simulink model "usmc2"  (R2020b)
settings: Solver=VariableStepAuto  StartTime=0.0  StopTime=10  RelTol=1e-3
settings Model: Creator=Lenovo  LastModifiedBy=Lenovo

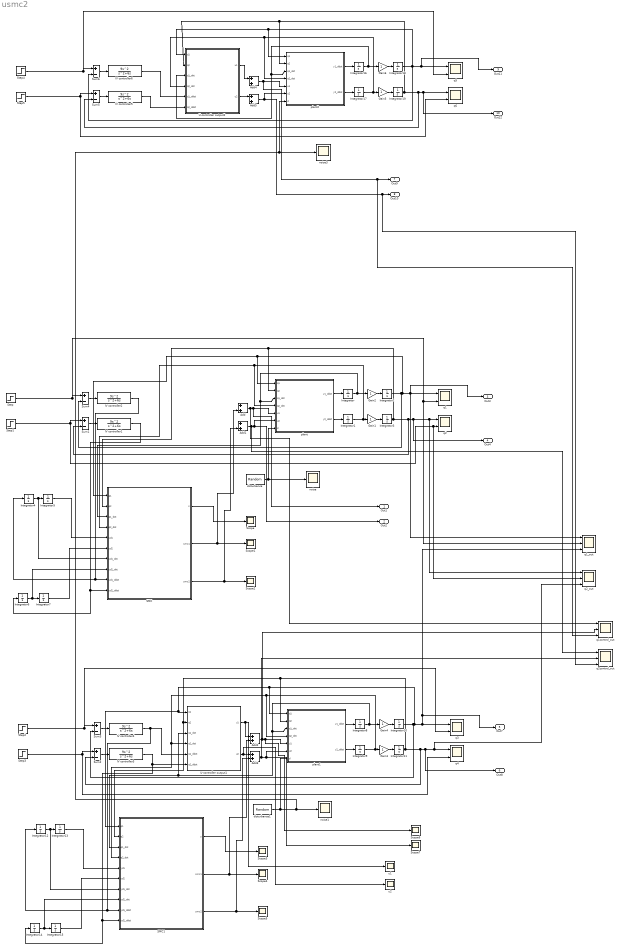
== system usmc2 ==
  Add{,1..5} (6 alike) : Sum
  Gain{1..6} (6 alike) : Gain
  IV controller{1..6} (6 alike) : TransferFcn  Numerator=[9 0 0]  Denominator=[1 6 0]
  Integrator{,1..19} (20 alike) : Integrator
  SMC : MATLAB Function  TreatAsAtomicUnit=on
  SMC1 : MATLAB Function  TreatAsAtomicUnit=on
  Scope{,1..7} (8 alike) : Scope
  Step : Step  After=3  SampleTime=0.001
  Step1 : Step  After=2  SampleTime=0.001
  Step2 : Step  After=3  SampleTime=0.001
  Step3 : Step  After=2  SampleTime=0.001
  Step4 : Step  After=3  SampleTime=0.001
  Step5 : Step  After=2  SampleTime=0.001
  Sum{1..6} (6 alike) : Sum  Inputs=|+-
  U-controller output1 : MATLAB Function  TreatAsAtomicUnit=on
  U-controller output2 : MATLAB Function  TreatAsAtomicUnit=on
  disturbance : UniformRandomNumber  Minimum=-10  Maximum=10  SampleTime=0.01
  disturbance1 : UniformRandomNumber  Minimum=-10  Maximum=10  SampleTime=0.01
  noise : Scope
  noise1 : Scope
  noise3 : Scope
  plant : MATLAB Function  TreatAsAtomicUnit=on
  plant1 : MATLAB Function  TreatAsAtomicUnit=on
  plant2 : MATLAB Function  TreatAsAtomicUnit=on
  q{1..6} (6 alike) : Scope  NumInputPorts=2
  q1_out : Scope  NumInputPorts=3
  q1control_out : Scope  NumInputPorts=3
  q2_out : Scope  NumInputPorts=3
  q2control_out : Scope  NumInputPorts=3
  u1 : Scope
  u2 : Scope
  Out1 : Outport  VectorParamsAs1DForOutWhenUnconnected=off
  Out2 : Outport  Port=2  VectorParamsAs1DForOutWhenUnconnected=off
  Out3 : Outport  Port=3  VectorParamsAs1DForOutWhenUnconnected=off
  Out4 : Outport  Port=4  VectorParamsAs1DForOutWhenUnconnected=off
  Out7 : Outport  Port=5  VectorParamsAs1DForOutWhenUnconnected=off
  Out8 : Outport  Port=6  VectorParamsAs1DForOutWhenUnconnected=off
  Out9 : Outport  Port=7  VectorParamsAs1DForOutWhenUnconnected=off
  Out10 : Outport  Port=8  VectorParamsAs1DForOutWhenUnconnected=off
  Out11 : Outport  Port=9  VectorParamsAs1DForOutWhenUnconnected=off
  Out12 : Outport  Port=10  VectorParamsAs1DForOutWhenUnconnected=off
  wires:
  Add5/1 -> q2control_out/3, Out10/1, plant2/6(u2)
  Integrator8/1 -> Gain4/1, SMC1/3(q1_dot), U-controller output1/3(q1_dot), plant1/3(q1_dot)
  Integrator16/1 -> Gain6/1, U-controller output2/3(q1_dot), plant2/3(q1_dot)
  Gain6/1 -> Integrator18/1
  plant2/1(y1_ddot) -> Integrator16/1
  Integrator10/1 -> q1_out/3, Out7/1, q3/1, SMC1/1(q1), U-controller output1/1(q1), plant1/1(q1), Sum3/2
  Integrator12/1 -> SMC1/7(yd1_dot), Integrator13/1
  Integrator14/1 -> SMC1/8(yd2_dot), Integrator15/1
  Integrator18/1 -> Out11/1, q5/1, U-controller output2/1(q1), plant2/1(q1), Sum6/2
  Add1/1 -> q2control_out/1, Out2/1, plant/6(u2)
  Integrator19/1 -> Out12/1, q6/1, Sum5/2, U-controller output2/2(q2), plant2/2(q2)
  U-controller output2/2(u2) -> Add5/1
  IV controller3/1 -> Integrator14/1, SMC1/10(yd2_ddot), U-controller output1/6(q2_ddot)
  plant/2(y2_ddot) -> Integrator1/1
  U-controller output2/1(u1) -> Add4/1
  plant2/2(y2_ddot) -> Integrator17/1
  Integrator9/1 -> U-controller output1/4(q2_dot), SMC1/4(q2_dot), plant1/4(q2_dot), Gain3/1
  plant1/1(y1_ddot) -> Integrator8/1
  IV controller6/1 -> U-controller output2/5(q1_ddot)
  disturbance1/1 -> plant1/7(d), plant2/7(d), noise3/1, noise1/1
  Step4/1 -> q5/2, Sum6/1
  Gain5/1 -> Integrator19/1
  Step5/1 -> q6/2, Sum5/1
  IV controller5/1 -> U-controller output2/6(q2_ddot)
  Gain1/1 -> Integrator3/1
  Sum6/1 -> IV controller6/1
  Gain3/1 -> Integrator11/1
  Sum2/1 -> IV controller3/1
  Step1/1 -> q2_out/2, q2/2, Sum1/1
  Gain2/1 -> Integrator2/1
  Sum4/1 -> IV controller2/1
  Step2/1 -> q3/2, Sum3/1
  Integrator2/1 -> q1_out/1, Out3/1, q1/1, SMC/1(q1), plant/1(q1), Sum4/2
  Sum3/1 -> IV controller4/1
  U-controller output1/1(u1) -> u1/1, Add2/1
  Add4/1 -> q1control_out/3, Out9/1, plant2/5(u1)
  Integrator1/1 -> SMC/4(q2_dot), plant/4(q2_dot), Gain1/1
  Sum1/1 -> IV controller1/1
  SMC/3(smc2) -> Add1/2, Scope2/1
  IV controller1/1 -> Integrator6/1, SMC/10(yd2_ddot)
  Integrator3/1 -> Out4/1, q2_out/1, q2/1, Sum1/2, SMC/2(q2), plant/2(q2)
  Add2/1 -> q1control_out/2, Scope6/1, plant1/5(u1)
  Sum5/1 -> IV controller5/1
  plant/1(y1_ddot) -> Integrator/1
  disturbance/1 -> plant/7(d), noise/1
  Integrator/1 -> Gain2/1, SMC/3(q1_dot), plant/3(q1_dot)
  U-controller output1/2(u2) -> u2/1, Add3/1
  Integrator5/1 -> SMC/5(yd1)
  IV controller2/1 -> Integrator4/1, SMC/9(yd1_ddot)
  Integrator4/1 -> SMC/7(yd1_dot), Integrator5/1
  Integrator6/1 -> SMC/8(yd2_dot), Integrator7/1
  Step3/1 -> q4/2, Sum2/1
  plant1/2(y2_ddot) -> Integrator9/1
  Integrator13/1 -> SMC1/5(yd1)
  SMC/2(smc1) -> Add/2, Scope1/1
  SMC1/3(smc2) -> Add3/2, Scope5/1
  SMC1/2(smc1) -> Add2/2, Scope4/1
  Gain4/1 -> Integrator10/1
  Integrator7/1 -> SMC/6(yd2)
  Integrator11/1 -> Out8/1, q2_out/3, q4/1, Sum2/2, SMC1/2(q2), U-controller output1/2(q2), plant1/2(q2)
  Step/1 -> q1_out/2, q1/2, Sum4/1
  IV controller4/1 -> Integrator12/1, SMC1/9(yd1_ddot), U-controller output1/5(q1_ddot)
  SMC/1(s) -> Scope/1
  Add3/1 -> Scope7/1, plant1/6(u2), q2control_out/2
  SMC1/1(s) -> Scope3/1
  Integrator15/1 -> SMC1/6(yd2)
  Add/1 -> q1control_out/1, Out1/1, plant/5(u1)
  Integrator17/1 -> U-controller output2/4(q2_dot), plant2/4(q2_dot), Gain5/1

== matlab function usmc2/plant2 ==
  data: q1 input; y1_ddot output; q2 input; q1_dot input; q2_dot input; y2_ddot output; u1 input; u2 input; d input
function [y1_ddot, y2_ddot] = fcn(q1, q2, q1_dot, q2_dot, u1, u2, d)

m1 = 1; m2 = 1;
l1 = 1; l2 = 1;
g = 9.8;
c2 = cos(q2);
s2 = sin(q2);
h = -0.5*m2*l1*l2*s2;
c1 = cos(q1);
c2 = cos(q2);
c12 = cos(q1+q2);


H = [1/3*m1*l1*l1+m2*l1*l1+1/3*m2*l2*l2+m2*l1*l2*c2, 1/3*m2*l2*l2+0.5*m2*l1*l2*c2;
    1/3*m2*l2*l2+1/2*m2*l1*l2*c2, 1/3*m2*l2*l2];

C = [h*q2_dot, h*(q1_dot+q2_dot);
     -h*q1_dot, 0];
 
G = [0.5*m1*g*l1*c1+m2*g*l1*c1+0.5*m2*g*l2*c12;
     0.5*m2*g*l2*c12];

output = inv(H) * ( [u1;u2] - C * [q1_dot;q2_dot] - G - d);

%%%%%% d means disturbance
y1_ddot = output(1,1);
y2_ddot = output(2,1);

== matlab function usmc2/SMC ==
  data: q1 input; s output; q2 input; q1_dot input; q2_dot input; smc1 output; yd1 input; yd2 input; yd1_dot input; yd2_dot input; yd1_ddot input; yd2_ddot input; smc2 output
function [s,smc1,smc2] = fcn(q1, q2, q1_dot, q2_dot, yd1,yd2,yd1_dot,yd2_dot,yd1_ddot,yd2_ddot)

m1 = 1; m2 = 1;
l1 = 1; l2 = 1;
g = 9.8;
c2 = cos(q2);
s2 = sin(q2);
h = -0.5*m2*l1*l2*s2;
c1 = cos(q1);
c2 = cos(q2);
c12 = cos(q1+q2);


H = [1/3*m1*l1*l1+m2*l1*l1+1/3*m2*l2*l2+m2*l1*l2*c2, 1/3*m2*l2*l2+0.5*m2*l1*l2*c2;
    1/3*m2*l2*l2+1/2*m2*l1*l2*c2, 1/3*m2*l2*l2];

C = [h*q2_dot, h*(q1_dot+q2_dot);
     -h*q1_dot, 0];
 
G = [0.5*m1*g*l1*c1+m2*g*l1*c1+0.5*m2*g*l2*c12;
     0.5*m2*g*l2*c12];

 
%%% smc
c1 = 10; c2 = 10; eita = 20;


z1 = [q1-yd1;q2-yd2];
z1_dot = [q1_dot-yd1_dot;q2_dot-yd2_dot];
z2 = c1 .* z1 + z1_dot;

%%%% sliding variable
s = z2;
sgn = s ./ (abs(s)+0.01);

%%%% control output
output = C * [q1_dot;q2_dot] + G + H * (-c1.*z1_dot+[yd1_ddot;yd2_ddot]-c2.*z2-z1) -eita.*sgn;

smc1 = output(1,1);
smc2 = output(2,1);

== matlab function usmc2/plant ==
  data: q1 input; y1_ddot output; q2 input; q1_dot input; q2_dot input; y2_ddot output; u1 input; u2 input; d input
function [y1_ddot, y2_ddot] = fcn(q1, q2, q1_dot, q2_dot, u1, u2, d)

m1 = 1; m2 = 1;
l1 = 1; l2 = 1;
g = 9.8;
c2 = cos(q2);
s2 = sin(q2);
h = -0.5*m2*l1*l2*s2;
c1 = cos(q1);
c2 = cos(q2);
c12 = cos(q1+q2);


H = [1/3*m1*l1*l1+m2*l1*l1+1/3*m2*l2*l2+m2*l1*l2*c2, 1/3*m2*l2*l2+0.5*m2*l1*l2*c2;
    1/3*m2*l2*l2+1/2*m2*l1*l2*c2, 1/3*m2*l2*l2];

C = [h*q2_dot, h*(q1_dot+q2_dot);
     -h*q1_dot, 0];
 
G = [0.5*m1*g*l1*c1+m2*g*l1*c1+0.5*m2*g*l2*c12;
     0.5*m2*g*l2*c12];

output = inv(H) * ( [u1;u2] - C * [q1_dot;q2_dot] - G - d);

%%%%%% d means disturbance
y1_ddot = output(1,1);
y2_ddot = output(2,1);

== matlab function usmc2/SMC1 ==
  data: q1 input; s output; q2 input; q1_dot input; q2_dot input; smc1 output; yd1 input; yd2 input; yd1_dot input; yd2_dot input; yd1_ddot input; yd2_ddot input; smc2 output
function [s,smc1,smc2] = fcn(q1, q2, q1_dot, q2_dot, yd1,yd2,yd1_dot,yd2_dot,yd1_ddot,yd2_ddot)

m1 = 1; m2 = 1;
l1 = 1; l2 = 1;
g = 9.8;
c2 = cos(q2);
s2 = sin(q2);
h = -0.5*m2*l1*l2*s2;
c1 = cos(q1);
c2 = cos(q2);
c12 = cos(q1+q2);


H = [1/3*m1*l1*l1+m2*l1*l1+1/3*m2*l2*l2+m2*l1*l2*c2, 1/3*m2*l2*l2+0.5*m2*l1*l2*c2;
    1/3*m2*l2*l2+1/2*m2*l1*l2*c2, 1/3*m2*l2*l2];

C = [h*q2_dot, h*(q1_dot+q2_dot);
     -h*q1_dot, 0];
 
G = [0.5*m1*g*l1*c1+m2*g*l1*c1+0.5*m2*g*l2*c12;
     0.5*m2*g*l2*c12];

 
%%% smc
c1 = 10; c2 = 10; eita = 20;


z1 = [q1-yd1;q2-yd2];
z1_dot = [q1_dot-yd1_dot;q2_dot-yd2_dot];
z2 = c1 .* z1 + z1_dot;

%%%% sliding variable
s = z2;
sgn = s ./ (abs(s)+0.01);

%%%% control output
output = C * [q1_dot;q2_dot] + G + H * (-c1.*z1_dot+[yd1_ddot;yd2_ddot]-c2.*z2-z1) -eita.*sgn;

smc1 = output(1,1);
smc2 = output(2,1);

== matlab function usmc2/U-controller output1 ==
  data: q1 input; u1 output; q2 input; q1_dot input; q2_dot input; u2 output; q1_ddot input; q2_ddot input
function [u1, u2] = fcn(q1, q2, q1_dot, q2_dot, q1_ddot, q2_ddot)

%%%%%%%%% Variables %%%%%%%%%%
m1 = 1; m2 = 1;
l1 = 1; l2 = 1;
g = 9.8;
c2 = cos(q2);
s2 = sin(q2);
h = -0.5*m2*l1*l2*s2;
c1 = cos(q1);
c2 = cos(q2);
co12 = cos(q1+q2);

y1_dot = q1_dot; y2_dot = q2_dot;
y1_ddot = q1_ddot; y2_ddot = q2_ddot;

%%%%%%%%% Matrix Calculation %%%%%%%%%%
H = [1/3*m1*l1*l1+m2*l1*l1+1/3*m2*l2*l2+m2*l1*l2*c2, 1/3*m2*l2*l2+0.5*m2*l1*l2*c2;
    1/3*m2*l2*l2+1/2*m2*l1*l2*c2, 1/3*m2*l2*l2];

C = [h*q2_dot, h*(q1_dot+q2_dot);
                      -h*q1_dot, 0];
c11 = C(1,1); c12 = C(1,2); c21 = C(2,1); c22 = C(2,2);                  


G = [0.5*m1*g*l1*c1+m2*g*l1*c1+0.5*m2*g*l2*co12;
     0.5*m2*g*l2*co12];
g1 = G(1,1); g2 = G(2,1);


M_ = inv(H);
m_11 = M_(1,1); m_12 = M_(1,2); m_21 = M_(2,1); m_22 = M_(2,2);

%%%%%%%%%% U-model output %%%%%%%%%%%
temp1 = -c11 * y1_dot - c12 * y2_dot - g1;
temp2 = -c21 * y1_dot - c22 * y2_dot - g2;

u1 = (m_22/m_12*y1_ddot-y2_ddot) / (m_22/m_12*m_11-m_21) - temp1;
u2 = (m_21/m_11*y1_ddot-y2_ddot) / (m_21/m_11*m_12-m_22) - temp2;

== matlab function usmc2/plant1 ==
  data: q1 input; y1_ddot output; q2 input; q1_dot input; q2_dot input; y2_ddot output; u1 input; u2 input; d input
function [y1_ddot, y2_ddot] = fcn(q1, q2, q1_dot, q2_dot, u1, u2, d)

m1 = 1; m2 = 1;
l1 = 1; l2 = 1;
g = 9.8;
c2 = cos(q2);
s2 = sin(q2);
h = -0.5*m2*l1*l2*s2;
c1 = cos(q1);
c2 = cos(q2);
c12 = cos(q1+q2);


H = [1/3*m1*l1*l1+m2*l1*l1+1/3*m2*l2*l2+m2*l1*l2*c2, 1/3*m2*l2*l2+0.5*m2*l1*l2*c2;
    1/3*m2*l2*l2+1/2*m2*l1*l2*c2, 1/3*m2*l2*l2];

C = [h*q2_dot, h*(q1_dot+q2_dot);
     -h*q1_dot, 0];
 
G = [0.5*m1*g*l1*c1+m2*g*l1*c1+0.5*m2*g*l2*c12;
     0.5*m2*g*l2*c12];


output = inv(H) * ( [u1;u2] - C * [q1_dot;q2_dot] - G - d);

%%%%%% d means disturbance
y1_ddot = output(1,1);
y2_ddot = output(2,1);

== matlab function usmc2/U-controller output2 ==
  data: q1 input; u1 output; q2 input; q1_dot input; q2_dot input; u2 output; q1_ddot input; q2_ddot input
function [u1, u2] = fcn(q1, q2, q1_dot, q2_dot, q1_ddot, q2_ddot)

%%%%%%%%% Variables %%%%%%%%%%
m1 = 1; m2 = 1;
l1 = 1; l2 = 1;
g = 9.8;
c2 = cos(q2);
s2 = sin(q2);
h = -0.5*m2*l1*l2*s2;
c1 = cos(q1);
c2 = cos(q2);
co12 = cos(q1+q2);

y1_dot = q1_dot; y2_dot = q2_dot;
y1_ddot = q1_ddot; y2_ddot = q2_ddot;

%%%%%%%%% Matrix Calculation %%%%%%%%%%
H = [1/3*m1*l1*l1+m2*l1*l1+1/3*m2*l2*l2+m2*l1*l2*c2, 1/3*m2*l2*l2+0.5*m2*l1*l2*c2;
    1/3*m2*l2*l2+1/2*m2*l1*l2*c2, 1/3*m2*l2*l2];

C = [h*q2_dot, h*(q1_dot+q2_dot);
                      -h*q1_dot, 0];
c11 = C(1,1); c12 = C(1,2); c21 = C(2,1); c22 = C(2,2);                  


G = [0.5*m1*g*l1*c1+m2*g*l1*c1+0.5*m2*g*l2*co12;
     0.5*m2*g*l2*co12];
g1 = G(1,1); g2 = G(2,1);


M_ = inv(H);
m_11 = M_(1,1); m_12 = M_(1,2); m_21 = M_(2,1); m_22 = M_(2,2);

%%%%%%%%%% U-model output %%%%%%%%%%%
temp1 = -c11 * y1_dot - c12 * y2_dot - g1;
temp2 = -c21 * y1_dot - c22 * y2_dot - g2;

u1 = (m_22/m_12*y1_ddot-y2_ddot) / (m_22/m_12*m_11-m_21) - temp1;
u2 = (m_21/m_11*y1_ddot-y2_ddot) / (m_21/m_11*m_12-m_22) - temp2;
